simulink model "controller"  (R2017b)
settings: Solver=FixedStepDiscrete  StartTime=0.0  StopTime=100  FixedStep=dt  RelTol=1e-3
values from neighbouring files (symbols this model uses):
  d = 0.15    [extendedKalman.m]    (also in extendedKalmanFilter.m; plant.m = 0.24; runV3.m; runpathfollower.m)
  dt = 0.1    [extendedKalmanFilter.m]    (also in matlab.mat; runV3.m; rungen.m; runpathfollower.m)
  k1 = 8    [runpathfollower.m]    (also in runpathplanner.m = 1)
  k2 = 1    [runpathfollower.m]    (also in runpathplanner.m)
  pxi = 2    [runpathfollower.m]    (also in runpathplanner.m = 0)
  pyi = 2    [runpathfollower.m]    (also in runpathplanner.m)
  velocity = 0.3    [runpathfollower.m]    (also in runpathplanner.m)
  xi0 = [0 0 0 0 0 0 0 0]    [matlab.mat]    (also in runV3.m = [0 0 0 0 0 0 0 0]'; runpathfollower.m = [xi,yi,0,0,0,0,theta_mi,0]'; runpathplanner.m = [xi,yi,0,0,0,0,theta_mi,0]')
libraries: simulink x1
settings Model: Creator=nisha  LastModifiedBy=nisha

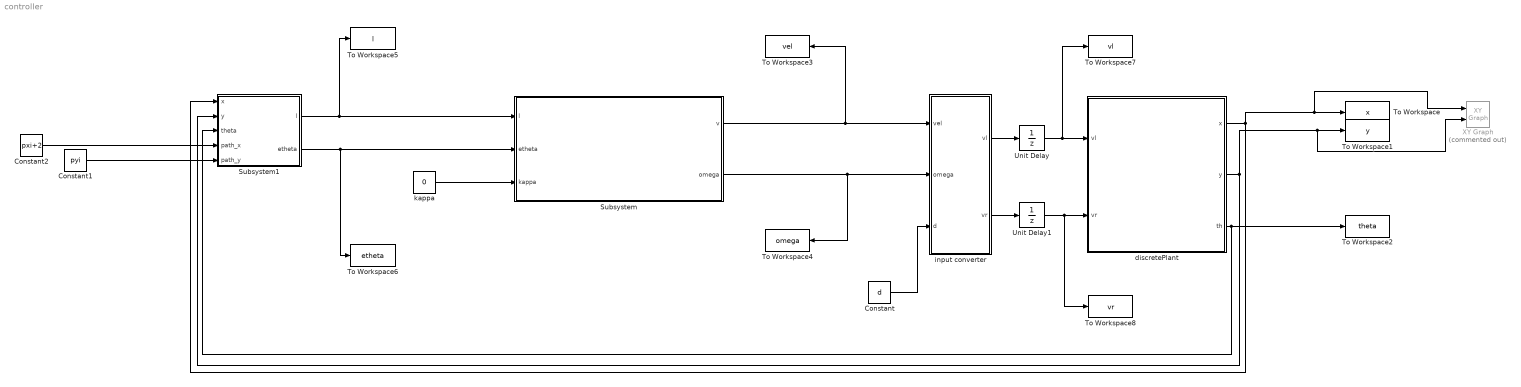
== system controller ==
  Constant : Constant  Value=d
  Constant1 : Constant  Value=pyi
  Constant2 : Constant  Value=pxi+2
  Subsystem : Subsystem
  Subsystem1 : Subsystem
  To Workspace : ToWorkspace  VariableName=x  SampleTime=-1
  To Workspace1 : ToWorkspace  VariableName=y  SampleTime=-1
  To Workspace2 : ToWorkspace  VariableName=theta  SampleTime=-1
  To Workspace3 : ToWorkspace  VariableName=vel  SampleTime=-1
  To Workspace4 : ToWorkspace  VariableName=omega  SampleTime=-1
  To Workspace5 : ToWorkspace  VariableName=l  SampleTime=-1
  To Workspace6 : ToWorkspace  VariableName=etheta  SampleTime=-1
  To Workspace7 : ToWorkspace  VariableName=vl  SampleTime=-1
  To Workspace8 : ToWorkspace  VariableName=vr  SampleTime=-1
  Unit Delay : UnitDelay  SampleTime=-1
  Unit Delay1 : UnitDelay  SampleTime=-1
  XY Graph : simulink/Sinks/XY Graph  Commented=on  xmin=-1  xmax=10  ymin=-1  ymax=1  st=-1
  discretePlant : Subsystem
  input converter : MATLAB Function  TreatAsAtomicUnit=on
  kappa : Constant  Value=0
  wires:
  input converter/2(vr) -> Unit Delay1/1
  input converter/1(vl) -> Unit Delay/1
  Constant/1 -> input converter/3(d)
  Subsystem/1(v) -> To Workspace3/1, input converter/1(vel)
  Subsystem/2(omega) -> input converter/2(omega), To Workspace4/1
  Subsystem1/1(l) -> To Workspace5/1, Subsystem/1(l)
  Subsystem1/2(etheta) -> To Workspace6/1, Subsystem/2(etheta)
  kappa/1 -> Subsystem/3(kappa)
  Constant1/1 -> Subsystem1/5(path_y)
  Constant2/1 -> Subsystem1/4(path_x)
  discretePlant/3(th) -> Subsystem1/3(theta), To Workspace2/1
  discretePlant/2(y) -> Subsystem1/2(y), XY Graph/2, To Workspace1/1
  Unit Delay/1 -> To Workspace7/1, discretePlant/1(vl)
  Unit Delay1/1 -> To Workspace8/1, discretePlant/2(vr)
  discretePlant/1(x) -> Subsystem1/1(x), XY Graph/1, To Workspace/1

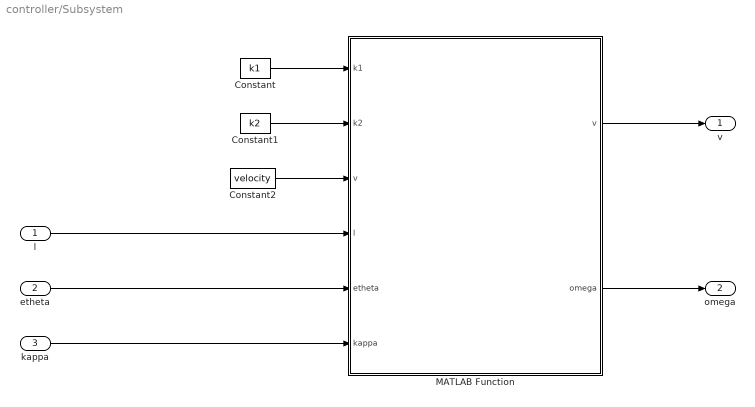
== system controller/Subsystem ==
  l : Inport
  etheta : Inport  Port=2
  kappa : Inport  Port=3
  Constant : Constant  Value=k1
  Constant1 : Constant  Value=k2
  Constant2 : Constant  Value=velocity
  MATLAB Function : MATLAB Function  TreatAsAtomicUnit=on
  v : Outport
  omega : Outport  Port=2
  wires:
  Constant/1 -> MATLAB Function/1(k1)
  Constant1/1 -> MATLAB Function/2(k2)
  Constant2/1 -> MATLAB Function/3("v ")
  l/1 -> MATLAB Function/4(l)
  etheta/1 -> MATLAB Function/5(etheta)
  kappa/1 -> MATLAB Function/6(kappa)
  MATLAB Function/1(v) -> v/1
  MATLAB Function/2(omega) -> omega/1

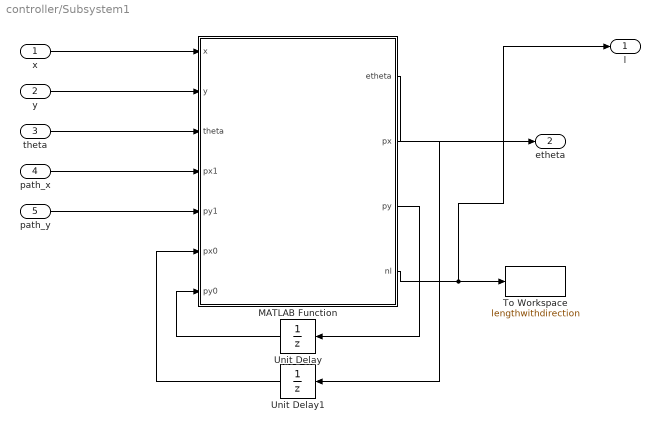
== system controller/Subsystem1 ==
  x : Inport
  y : Inport  Port=2
  theta : Inport  Port=3
  path_x : Inport  Port=4
  path_y : Inport  Port=5
  MATLAB Function : MATLAB Function  TreatAsAtomicUnit=on
  To Workspace : ToWorkspace  VariableName=lengthwithdirection  SampleTime=-1
  Unit Delay : UnitDelay  InitialCondition=pyi  SampleTime=-1
  Unit Delay1 : UnitDelay  InitialCondition=pxi  SampleTime=-1
  l : Outport
  etheta : Outport  Port=2
  wires:
  x/1 -> MATLAB Function/1(x)
  y/1 -> MATLAB Function/2(y)
  path_x/1 -> MATLAB Function/4(px1)
  theta/1 -> MATLAB Function/3(theta)
  MATLAB Function/1(etheta) -> etheta/1
  MATLAB Function/4(nl) -> l/1, To Workspace/1
  MATLAB Function/2(px) -> Unit Delay1/1
  MATLAB Function/3(py) -> Unit Delay/1
  path_y/1 -> MATLAB Function/5(py1)
  Unit Delay/1 -> MATLAB Function/7(py0)
  Unit Delay1/1 -> MATLAB Function/6(px0)

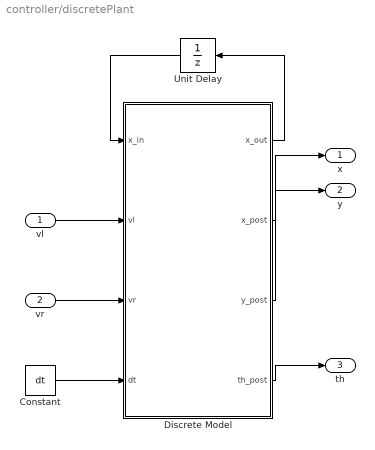
== system controller/discretePlant ==
  vl : Inport
  vr : Inport  Port=2
  Constant : Constant  Value=dt
  Discrete Model : MATLAB Function  TreatAsAtomicUnit=on
  Unit Delay : UnitDelay  InitialCondition=xi0  SampleTime=-1
  x : Outport
  y : Outport  Port=2
  th : Outport  Port=3
  wires:
  vl/1 -> Discrete Model/2(vl)
  Discrete Model/1(x_out) -> Unit Delay/1
  Unit Delay/1 -> Discrete Model/1(x_in)
  vr/1 -> Discrete Model/3(vr)
  Discrete Model/2(x_post) -> x/1
  Discrete Model/3(y_post) -> y/1
  Discrete Model/4(th_post) -> th/1
  Constant/1 -> Discrete Model/4(dt)

== matlab function controller/Subsystem/MATLAB Function ==
  data: k1 input; v output; k2 input; v input; l input; etheta input; kappa input; omega output
function [v,omega] = fcn(k1, k2, v, l, etheta, kappa)
omega= kappa*cos(etheta)*v/(1-kappa*l)-k1*l*v*sin(etheta)/etheta-k2*etheta;

== matlab function controller/input converter ==
  data: vel input; vl output; omega input; d input; vr output
function [vl, vr] = fcn(vel, omega,d)
vr=vel +d/2*omega;
vl=vel -d/2*omega;
end

== matlab function controller/Subsystem1/MATLAB Function ==
  data: x input; y input; theta input; px1 input; etheta output; py1 input; px output; py output; px0 input; py0 input; nl output
function [ etheta,px,py,nl] = fcn(x,y,theta,px1,py1,px0,py0)
v=[px1-px0,py1-py0];
w=[x-px0,y-py0];
px=px0; py=py0;

theta_r=acos(dot(v,[1,0])/norm(v));
rot=[cos(theta_r) -sin(theta_r)
    sin(theta_r) cos(theta_r)];
length=rot*w';
nl=dot(length,[0; 1]);
etheta=theta-theta_r;

== matlab function controller/discretePlant/Discrete Model ==
  data: x_in input; x_out output; vl input; vr input; x_post output; y_post output; th_post output; dt input
function [x_out,x_post,y_post,th_post]         = fcn(x_in,vl, vr,dt)

d=0.15;
x=x_in(1); y=x_in(2); dx=x_in(3);dy=x_in(4);ddx=x_in(5);ddy=x_in(6); phi=x_in(7); dphi=x_in(8);
th=phi+0.5*dphi*dt;
x_out = ...
[x + dx*dt + ddx*dt^2/2
 y + dy*dt + ddy*dt^2/2
 (vl+vr)/2*cos(th)+ddx*dt
 (vl+vr)/2*sin(th)+ddy*dt
 ddx
 ddy
 phi + dphi*dt
 (vr-vl)/d];

x_post=x_out(1); y_post=x_out(2); th_post=x_out(7);
end
